simulink model "PT2_schwingfaehig_model"  (R2024a)
settings: Solver=ode45  StartTime=0.0  StopTime=20.0  FixedStep=1e-2  RelTol=1e-4  AbsTol=1e-4
undefined symbols (not defined in the file): den, Kp, lower_limit, num, Tn, Tv, upper_limit
settings Model: Creator=bhir  LastModifiedBy=Flo
settings SolverCC: AlgebraicLoopSolver=TrustRegion
settings DataIOCC: ReturnWorkspaceOutputs=off
settings DebuggingCC: UnconnectedInputMsg=warning  UnconnectedOutputMsg=warning  UnconnectedLineMsg=warning  ArithmeticOperatorsInVariantConditions=warning
settings SFSimCC: SimUseLocalCustomCode=off  CustomCodeUndefinedFunction=UseInterfaceOnly
settings RTWCC: RTWUseLocalCustomCode=off  GPUComputeCapability=3.5  DLArmComputeVersion=19.05
settings CodeAppCC: StateflowObjectComments=on

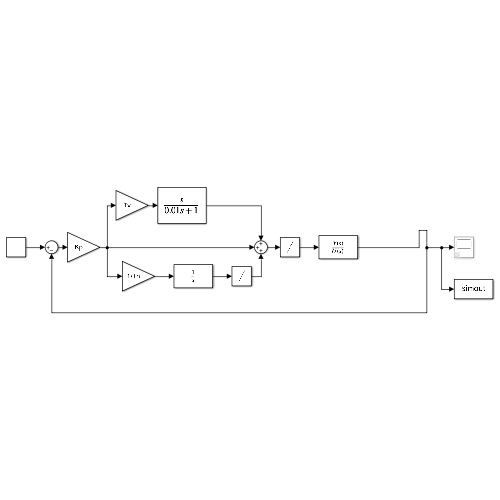
[thumbnail: Simulink's stored preview of the top-level diagram]
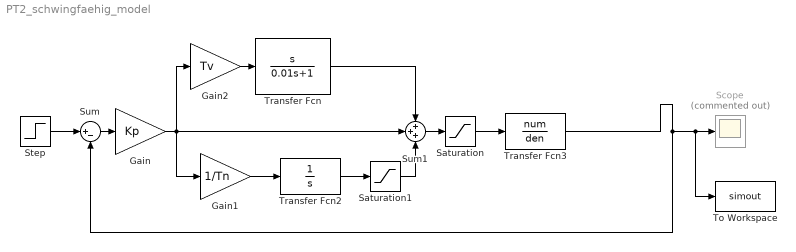
== system PT2_schwingfaehig_model ==
  Gain : Gain  Gain=Kp
  Gain1 : Gain  Gain=1/Tn
  Gain2 : Gain  Gain=Tv
  Saturation : Saturate  UpperLimit=upper_limit  LowerLimit=lower_limit
  Saturation1 : Saturate  UpperLimit=upper_limit  LowerLimit=lower_limit
  Scope : Scope  Commented=on
  Step : Step  Time=0  SampleTime=0
  Sum : Sum  Inputs=|+-
  Sum1 : Sum  Inputs=+++
  To Workspace : ToWorkspace  VariableName=simout  SaveFormat=Structure With Time  SampleTime=-1
  Transfer Fcn : TransferFcn  Numerator=[1 0]  Denominator=[0.01 1]
  Transfer Fcn2 : TransferFcn  Denominator=[1 0]
  Transfer Fcn3 : TransferFcn  Numerator=num  Denominator=den
  wires:
  Step/1 -> Sum/1
  Sum/1 -> Gain/1
  Gain1/1 -> Transfer Fcn2/1
  Sum1/1 -> Saturation/1
  Gain/1 -> Gain2/1, Sum1/2, Gain1/1
  Transfer Fcn/1 -> Sum1/1
  Gain2/1 -> Transfer Fcn/1
  Transfer Fcn3/1 -> Sum/2, To Workspace/1, Scope/1
  Saturation/1 -> Transfer Fcn3/1
  Transfer Fcn2/1 -> Saturation1/1
  Saturation1/1 -> Sum1/3
